simulink subsystem "BLDC_Motor_Sub2"  (R2020b)
settings: Solver=VariableStepAuto  StartTime=0.0  StopTime=10.0  RelTol=1e-3
libraries: fl_lib x29, nesl_utility x9, ee_lib x1
settings Model: Creator=Chrille Skog  LastModifiedBy=Chrille Skog

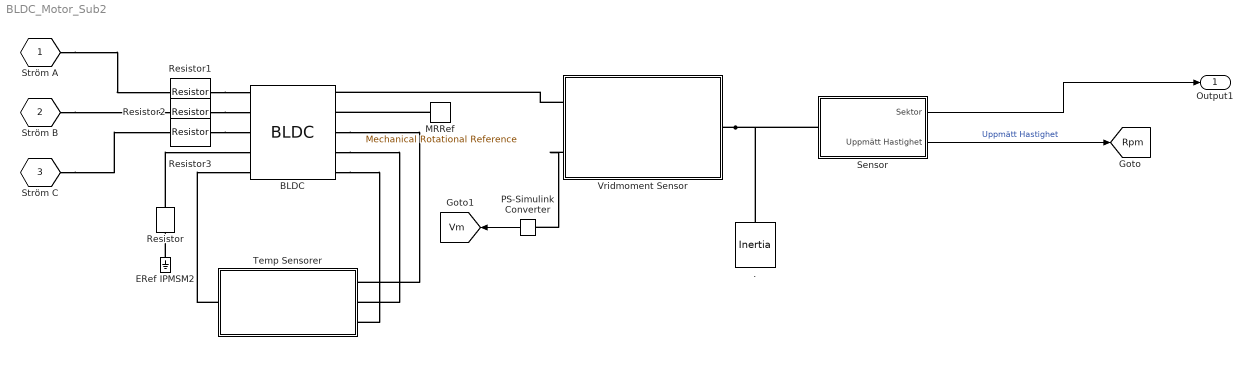
== system BLDC_Motor_Sub2 ==
  . : fl_lib/Mechanical/Rotational Elements/Inertia  inertia=2 kg*m^2  num_ports=foundation.enum.numPorts2.one  w_specify=off  w_priority=High  w=0 rpm  w_nominal_specify=off  w_nominal_unit=rad/s  w_nominal_value=1  t_specify=off  t_priority=High  t=0 N*m  t_nominal_specify=off  t_nominal_unit=N*m  t_nominal_value=1
      settings: SourceProductName=Foundation Library
  BLDC : ee_lib/Electromechanical/Permanent Magnet/BLDC  winding_type=ee.enum.statorconnection.wye  rotor_param=ee.enum.pmsm.backemf.trapezoidflux  pm_flux_linkage=0.05 Wb  theta_constant=120/3 deg  emf_max=9.6 V  DphiDtheta_tab=[0, -.1528, -.1528, .1528, .1528, 0] Wb/rad  back_emf_tab=[0, -9.6, -9.6, 9.6, 9.6, 0] V  rotor_angle_tab=[0, 7.5, 22.5, 37.5, 52.5, 60] deg  w_meas=600 rpm  nPolePairs=3  stator_param=ee.enum.statorparam.LdLqL0  machine_param=ee.enum.dqparameterization.constant  Ld=0.00022 H  Lq=0.00022 H  idVec=[-200, 0, 200] A  iqVec=[-200, 0, 200] A  LdMatrix=0.00022 * ones(3, 3) H  LqMatrix=0.00022 * ones(3, 3) H  L0=0.00016 H  Ls=0.0002 H  Lm=0 H  Ms=0.00002 H  Rs=0.0013 Ohm  zero_sequence=ee.enum.park.zerosequence.include  J=0 kg*m^2  lam=0.1 N*m/(rad/s)  axes_param=ee.enum.rotorangle.qaxis  i_d_specify=off  i_d_priority=None  i_d=0 A  i_d_nominal_specify=off  i_d_nominal_unit=A  i_d_nominal_value=1  i_q_specify=off  i_q_priority=None  i_q=0 A  i_q_nominal_specify=off  i_q_nominal_unit=A  i_q_nominal_value=1  torque_specify=off  torque_priority=None  torque=0 N*m  torque_nominal_specify=off  torque_nominal_unit=N*m  torque_nominal_value=1  angular_velocity_specify=off  angular_velocity_priority=High  angular_velocity=0 rpm  angular_velocity_nominal_specify=off  angular_velocity_nominal_unit=rpm  angular_velocity_nominal_value=1  angular_position_specify=off  angular_position_priority=High  angular_position=0 deg  angular_position_nominal_specify=off  angular_position_nominal_unit=deg  angular_position_nominal_value=1  loss_param=ee.enum.ironloss.none  losses_oc=[0, 0, 0] W  losses_sc=[0, 0, 0] W  f_losses=60 Hz  Isc_losses=95 A  Tmeas=298.15 K  alpha=3.93e-3 1/K  alpha_flux=-0.001 1/K  stator_thermal_mass=100 J/K  rotor_thermal_mass=200 J/K  Rm_percent_rotor=90  Rd_percent_rotor=30  temperatureA_specify=off  temperatureA_priority=High  temperatureA=25 degC  temperatureA_nominal_specify=off  temperatureA_nominal_unit=degC  temperatureA_nominal_value=1  temperatureB_specify=off  temperatureB_priority=High  temperatureB=25 degC  temperatureB_nominal_specify=off  temperatureB_nominal_unit=degC  temperatureB_nominal_value=1  temperatureC_specify=off  temperatureC_priority=High  temperatureC=25 degC  temperatureC_nominal_specify=off  temperatureC_nominal_unit=degC  temperatureC_nominal_value=1  temperatureR_specify=off  temperatureR_priority=High  temperatureR=25 degC  temperatureR_nominal_specify=off  temperatureR_nominal_unit=degC  temperatureR_nominal_value=1
      settings: SourceProductBaseCode=PS  InternalSimscapePortConfiguration="{\"Bottom\":[],\"Left\":[{\"id\":\"a\",\"label\":\"a\",\"type\":\"foundation.electrical.electrical\"},{\"id\":\"b\",\"label\":\"b\",\"type\":\"foundation.electrical.electrical\"},{\"id\":\"c\",\"label\":\"c\",\"type\":\"foundation.electrical.electrical\"},{\"id\":\"n\",\"label\":\"n\",\"type\":\"foundation.electrical.electrical\"},{\"id\":\"HR\",\"label\":\"HR\",\"type\":\"foundation.thermal.thermal\"}],\"Right\":[{\"id\":\"R\",\"label\":\"R\",\"type\":\"foundation.mechanical.rotational.rotational\"},{\"id\":\"C\",\"label\":\"C\",\"type\":\"foundation.mechanical.rotational.rotational\"},{\"id\":\"HA\",\"label\":\"HA\",\"type\":\"foundation.thermal.thermal\"},{\"id\":\"HB\",\"label\":\"HB\",\"type\":\"foundation.thermal.thermal\"},{\"id\":\"HC\",\"label\":\"HC\",\"type\":\"foundation.thermal.thermal\"}],\"Top\":[]}"
  ERef IPMSM2 : fl_lib/Electrical/Electrical Elements/Electrical Reference
  MRRef : fl_lib/Mechanical/Rotational Elements/Mechanical Rotational Reference
  PS-Simulink Converter : nesl_utility/PS-Simulink Converter  PhysicalDomain=network_engine_domain  SubClassName=ps_output  LeftPortType=input  RightPortType=output  PseudoPeriodic=off  Frequencies=[]  Unit=inherit  AffineConversion=off
  Resistor : fl_lib/Electrical/Electrical Elements/Resistor  R=1e9 Ohm  i_specify=off  i_priority=None  i=0 A  i_nominal_specify=off  i_nominal_unit=A  i_nominal_value=1  v_specify=off  v_priority=None  v=0 V  v_nominal_specify=off  v_nominal_unit=V  v_nominal_value=1
  Resistor1 : fl_lib/Electrical/Electrical Elements/Resistor  R=0 Ohm  i_specify=off  i_priority=None  i=0 A  i_nominal_specify=off  i_nominal_unit=A  i_nominal_value=1  v_specify=off  v_priority=None  v=0 V  v_nominal_specify=off  v_nominal_unit=V  v_nominal_value=1
  Resistor2 : fl_lib/Electrical/Electrical Elements/Resistor  R=0 Ohm  i_specify=off  i_priority=None  i=0 A  i_nominal_specify=off  i_nominal_unit=A  i_nominal_value=1  v_specify=off  v_priority=None  v=0 V  v_nominal_specify=off  v_nominal_unit=V  v_nominal_value=1
  Resistor3 : fl_lib/Electrical/Electrical Elements/Resistor  R=0 Ohm  i_specify=off  i_priority=None  i=0 A  i_nominal_specify=off  i_nominal_unit=A  i_nominal_value=1  v_specify=off  v_priority=None  v=0 V  v_nominal_specify=off  v_nominal_unit=V  v_nominal_value=1
  Sensor : Subsystem
  Temp Sensorer : Subsystem
  Vridmoment Sensor : Subsystem
  Ström A : PMIOPort  Tag=PMCPort  Side=Left
  Ström B : PMIOPort  Tag=PMCPort  Port=2  Side=Left
  Ström C : PMIOPort  Tag=PMCPort  Port=3  Side=Left
  Output1 : Outport
  tag scope: Rpm=global, Vm=global
  wires:
  Sensor/1(Sektor) -> Output1/1
  Sensor/2(Uppmätt Hastighet) -> [Rpm]  "Uppmätt Hastighet"
  PS-Simulink Converter/1 -> [Vm]
  connections:
  Vridmoment Sensor/RConn1 -- ./LConn1 -- Sensor/LConn1
  Ström B/RConn1 -- Resistor2/LConn1
  Resistor/LConn1 -- BLDC/LConn4
  Vridmoment Sensor/LConn1 -- BLDC/RConn1
  MRRef/LConn1 -- BLDC/RConn2
  BLDC/RConn4 -- Temp Sensorer/LConn2
  BLDC/RConn3 -- Temp Sensorer/LConn1
  Temp Sensorer/RConn1 -- BLDC/LConn5
  BLDC/RConn5 -- Temp Sensorer/LConn3
  ERef IPMSM2/LConn1 -- Resistor/RConn1
  Ström C/RConn1 -- Resistor3/LConn1
  Ström A/RConn1 -- Resistor1/LConn1
  Vridmoment Sensor/LConn2 -- PS-Simulink Converter/LConn1
  Resistor1/RConn1 -- BLDC/LConn1
  Resistor2/RConn1 -- BLDC/LConn2
  Resistor3/RConn1 -- BLDC/LConn3

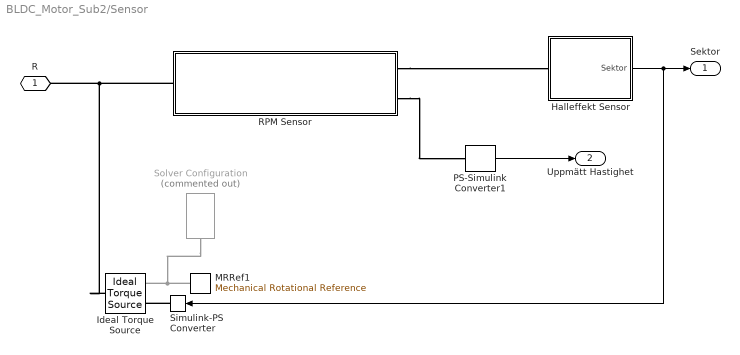
== system BLDC_Motor_Sub2/Sensor ==
  Halleffekt Sensor : Subsystem
  Ideal Torque Source : fl_lib/Mechanical/Mechanical Sources/Ideal Torque Source
  MRRef1 : fl_lib/Mechanical/Rotational Elements/Mechanical Rotational Reference
  PS-Simulink Converter1 : nesl_utility/PS-Simulink Converter  PhysicalDomain=network_engine_domain  SubClassName=ps_output  LeftPortType=input  RightPortType=output  PseudoPeriodic=off  Frequencies=[]  Unit=rpm  AffineConversion=off
  RPM Sensor : Subsystem
  Simulink-PS Converter : nesl_utility/Simulink-PS Converter  PhysicalDomain=network_engine_domain  SubClassName=ps_input  LeftPortType=input  RightPortType=output  PseudoPeriodic=off  Frequencies=[]  NoiseDistribution=none  NoiseParameters=[]  Unit=N*m  AffineConversion=off  FilteringAndDerivatives=provide  SimscapeFilterOrder=1  InputFilterTimeConstant=0.001  UdotUserProvided=0
  Solver Configuration : nesl_utility/Solver Configuration  Commented=on  PhysicalDomain=network_engine_domain  SubClassName=solver  LeftPortType=input  RightPortType=generic  Tones=[]  Harmonics=[]  SimulateNoise=off  Profile=off  UseLocalSampling=off  EnableSwitchedLinearOptims=on  FrequencyDomain=off  UseCCode=off  RelTol=0.001  AbsTol=1e-06  MinStep=1e-09  ToWorkspace=off  RevertToSquareIcSolve=off  NumHomotopyIterations=100  PhasorMode=off  PhasorModeNumHarmonics=1  DoDC=off  ResidualTolerance=1e-09  UseLocalSolver=on  LocalSolverChoice=NE_BACKWARD_EULER_ADVANCER  LocalSolverSampleTime=0.001  DoFixedCost=on  MaxNonlinIter=2  MaxModeIter=2  ComputeImpulses=off  ImpulseIterations=2  LinearAlgebra=auto  EquationFormulation=NE_TIME_EF  DelaysMemoryBudget=1024  AutomaticFiltering=on  FilteringTimeConstant=0.001  PartitionStorageMethod=AS_NEEDED  PartitionMemoryBudget=1024  PartitionMethod=FAST
  R : PMIOPort  Side=Left
  Sektor : Outport
  Uppmätt Hastighet : Outport  Port=2
  wires:
  PS-Simulink Converter1/1 -> Uppmätt Hastighet/1
  Halleffekt Sensor/1(Sektor) -> Simulink-PS Converter/1, Sektor/1
  connections:
  RPM Sensor/LConn1 -- R/RConn1 -- Ideal Torque Source/LConn1
  RPM Sensor/RConn2 -- PS-Simulink Converter1/LConn1
  RPM Sensor/RConn1 -- Halleffekt Sensor/LConn1
  Solver Configuration/RConn1 -- MRRef1/LConn1 -- Ideal Torque Source/RConn2
  Simulink-PS Converter/RConn1 -- Ideal Torque Source/RConn1

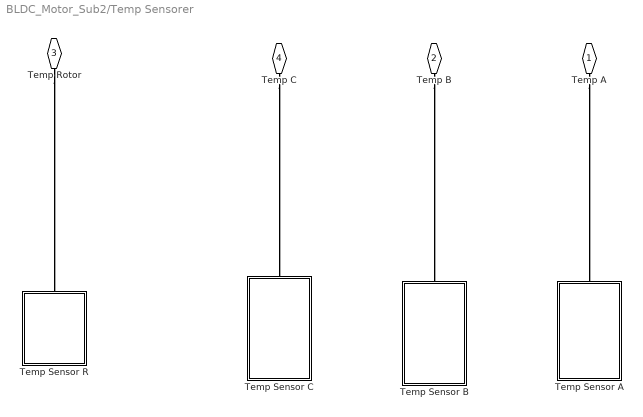
== system BLDC_Motor_Sub2/Temp Sensorer ==
  Temp Sensor A : Subsystem
  Temp Sensor B : Subsystem
  Temp Sensor C : Subsystem
  Temp Sensor R : Subsystem
  Temp A : PMIOPort  Side=Left
  Temp B : PMIOPort  Port=2  Side=Left
  "Temp Rotor " : PMIOPort  Port=3  Side=Right
  Temp C : PMIOPort  Port=4  Side=Left
  connections:
  Temp B/RConn1 -- Temp Sensor B/LConn1
  Temp A/RConn1 -- Temp Sensor A/LConn1
  Temp C/RConn1 -- Temp Sensor C/LConn1
  "Temp Rotor "/RConn1 -- Temp Sensor R/RConn1

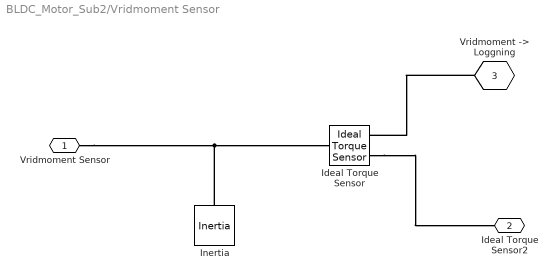
== system BLDC_Motor_Sub2/Vridmoment Sensor ==
  Ideal Torque Sensor : fl_lib/Mechanical/Mechanical Sensors/Ideal Torque Sensor
  Inertia : fl_lib/Mechanical/Rotational Elements/Inertia  inertia=0.01 kg*m^2  num_ports=foundation.enum.numPorts2.one  w_specify=off  w_priority=High  w=0 rad/s  w_nominal_specify=off  w_nominal_unit=rad/s  w_nominal_value=1  t_specify=off  t_priority=None  t=0 N*m  t_nominal_specify=off  t_nominal_unit=N*m  t_nominal_value=1
  Vridmoment Sensor : PMIOPort  Side=Left
  Ideal Torque Sensor2 : PMIOPort  Port=2  Side=Right
  "Vridmoment -> Loggning" : PMIOPort  Tag=PMCPort  Port=3  Side=Left
  connections:
  "Vridmoment -> Loggning"/RConn1 -- Ideal Torque Sensor/RConn2
  Ideal Torque Sensor/RConn1 -- Ideal Torque Sensor2/RConn1
  Vridmoment Sensor/RConn1 -- Ideal Torque Sensor/LConn1 -- Inertia/LConn1

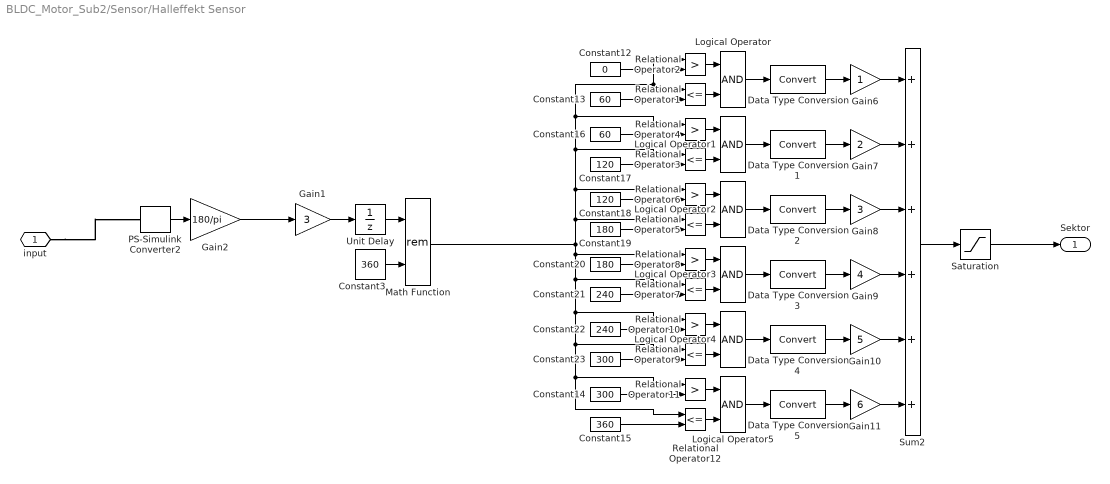
== system BLDC_Motor_Sub2/Sensor/Halleffekt Sensor ==
  Constant12 : Constant  Value=0
  Constant13 : Constant  Value=60
  Constant14 : Constant  Value=300
  Constant15 : Constant  Value=360
  Constant16 : Constant  Value=60
  Constant17 : Constant  Value=120
  Constant18 : Constant  Value=120
  Constant19 : Constant  Value=180
  Constant20 : Constant  Value=180
  Constant21 : Constant  Value=240
  Constant22 : Constant  Value=240
  Constant23 : Constant  Value=300
  Constant3 : Constant  Value=360
  Data Type Conversion{,1..5} (6 alike) : DataTypeConversion  SaturateOnIntegerOverflow=on  RndMeth=Zero
  Gain1 : Gain  Gain=3
  Gain10 : Gain  Gain=5  SaturateOnIntegerOverflow=on  OutDataTypeStr=Inherit: Same as input  ParamDataTypeStr=Inherit: Same as input
  Gain11 : Gain  Gain=6  SaturateOnIntegerOverflow=on  OutDataTypeStr=Inherit: Same as input  ParamDataTypeStr=Inherit: Same as input
  Gain2 : Gain  Gain=180/pi
  Gain6 : Gain  SaturateOnIntegerOverflow=on  OutDataTypeStr=Inherit: Same as input  ParamDataTypeStr=Inherit: Same as input
  Gain7 : Gain  Gain=2  SaturateOnIntegerOverflow=on  OutDataTypeStr=Inherit: Same as input  ParamDataTypeStr=Inherit: Same as input
  Gain8 : Gain  Gain=3  SaturateOnIntegerOverflow=on  OutDataTypeStr=Inherit: Same as input  ParamDataTypeStr=Inherit: Same as input
  Gain9 : Gain  Gain=4  SaturateOnIntegerOverflow=on  OutDataTypeStr=Inherit: Same as input  ParamDataTypeStr=Inherit: Same as input
  Logical Operator{,1..5} (6 alike) : Logic
  Math Function : Math  Operator=rem  SignedPower=on  SaturateOnIntegerOverflow=on
  PS-Simulink Converter2 : nesl_utility/PS-Simulink Converter  PhysicalDomain=network_engine_domain  SubClassName=ps_output  LeftPortType=input  RightPortType=output  PseudoPeriodic=off  Frequencies=[]  Unit=rad  AffineConversion=off
  Relational Operator{1,3,5,7,9,12} (6 alike) : RelationalOperator  Operator=<=  RndMeth=Nearest  InputSameDT=on
  Relational Operator{2,4,6,8,10..11} (6 alike) : RelationalOperator  Operator=>  RndMeth=Nearest  InputSameDT=on
  Saturation : Saturate  UpperLimit=6  LowerLimit=1
  Sum2 : Sum  Inputs=++++++  InputSameDT=on  SaturateOnIntegerOverflow=on  OutDataTypeStr=Inherit: Same as first input
  Unit Delay : UnitDelay  SampleTime=5.0e-5  HasFrameUpgradeWarning=on
  input : PMIOPort  Side=Left
  Sektor : Outport
  wires:
  Constant12/1 -> Relational Operator2/2
  Gain2/1 -> Gain1/1
  Math Function/1 -> Relational Operator2/1, Relational Operator1/1, Relational Operator4/1, Relational Operator3/1, Relational Operator6/1, Relational Operator5/1, Relational Operator12/1, Relational Operator11/1, Relational Operator9/1, Relational Operator10/1, Relational Operator7/1, Relational Operator8/1
  Relational Operator8/1 -> Logical Operator3/1
  Data Type Conversion5/1 -> Gain11/1
  Relational Operator7/1 -> Logical Operator3/2
  Logical Operator5/1 -> Data Type Conversion5/1
  Constant20/1 -> Relational Operator8/2
  Data Type Conversion1/1 -> Gain7/1
  Data Type Conversion2/1 -> Gain8/1
  Logical Operator2/1 -> Data Type Conversion2/1
  Constant18/1 -> Relational Operator6/2
  Relational Operator3/1 -> Logical Operator1/2
  Relational Operator4/1 -> Logical Operator1/1
  Logical Operator3/1 -> Data Type Conversion3/1
  Relational Operator9/1 -> Logical Operator4/2
  Data Type Conversion4/1 -> Gain10/1
  Relational Operator2/1 -> Logical Operator/1
  Relational Operator1/1 -> Logical Operator/2
  Sum2/1 -> Saturation/1
  Logical Operator/1 -> Data Type Conversion/1
  Constant19/1 -> Relational Operator5/2
  Constant16/1 -> Relational Operator4/2
  Constant17/1 -> Relational Operator3/2
  Relational Operator5/1 -> Logical Operator2/2
  Relational Operator6/1 -> Logical Operator2/1
  Gain10/1 -> Sum2/5
  Data Type Conversion3/1 -> Gain9/1
  Logical Operator1/1 -> Data Type Conversion1/1
  Relational Operator12/1 -> Logical Operator5/2
  Logical Operator4/1 -> Data Type Conversion4/1
  Constant21/1 -> Relational Operator7/2
  Constant22/1 -> Relational Operator10/2
  Gain8/1 -> Sum2/3
  Gain7/1 -> Sum2/2
  Data Type Conversion/1 -> Gain6/1
  Gain6/1 -> Sum2/1
  Relational Operator10/1 -> Logical Operator4/1
  PS-Simulink Converter2/1 -> Gain2/1
  Constant23/1 -> Relational Operator9/2
  Relational Operator11/1 -> Logical Operator5/1
  Constant13/1 -> Relational Operator1/2
  Constant3/1 -> Math Function/2
  Constant14/1 -> Relational Operator11/2
  Gain1/1 -> Unit Delay/1
  Gain9/1 -> Sum2/4
  Unit Delay/1 -> Math Function/1
  Gain11/1 -> Sum2/6
  Constant15/1 -> Relational Operator12/2
  Saturation/1 -> Sektor/1
  connections:
  input/RConn1 -- PS-Simulink Converter2/LConn1

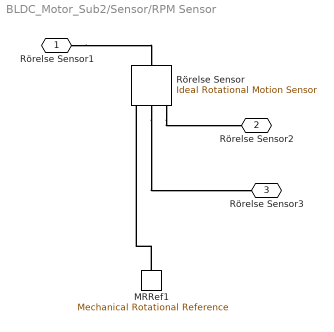
== system BLDC_Motor_Sub2/Sensor/RPM Sensor ==
  MRRef1 : fl_lib/Mechanical/Rotational Elements/Mechanical Rotational Reference
  Rörelse Sensor : fl_lib/Mechanical/Mechanical Sensors/Ideal Rotational Motion Sensor  wrap_angle=simscape.enum.onoff.off  offset=0 deg
      settings: SourceProductName=Foundation Library
  Rörelse Sensor1 : PMIOPort  Side=Left
  Rörelse Sensor2 : PMIOPort  Port=2  Side=Right
  Rörelse Sensor3 : PMIOPort  Port=3  Side=Right
  connections:
  Rörelse Sensor/RConn3 -- Rörelse Sensor2/RConn1
  MRRef1/LConn1 -- Rörelse Sensor/RConn1
  Rörelse Sensor1/RConn1 -- Rörelse Sensor/LConn1
  Rörelse Sensor/RConn2 -- Rörelse Sensor3/RConn1

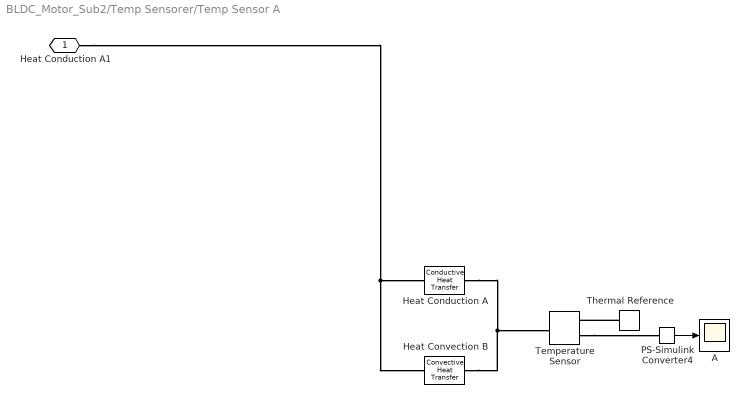
== system BLDC_Motor_Sub2/Temp Sensorer/Temp Sensor A ==
  A : Scope
  Heat Conduction A : fl_lib/Thermal/Thermal Elements/Conductive Heat Transfer  area=0.002 m^2  thickness=0.1 m  th_cond=80 W/(m*K)  T_specify=off  T_priority=None  T=0 K  T_nominal_specify=off  T_nominal_unit=K  T_nominal_value=1  Q_specify=off  Q_priority=None  Q=0 J/s  Q_nominal_specify=off  Q_nominal_unit=J/s  Q_nominal_value=1
      settings: SourceProductName=Foundation Library
  Heat Convection B : fl_lib/Thermal/Thermal Elements/Convective Heat Transfer  area=0.02 m^2  heat_tr_coeff=200 W/(m^2 * K)  T_specify=off  T_priority=None  T=0 K  T_nominal_specify=off  T_nominal_unit=K  T_nominal_value=1  Q_specify=off  Q_priority=None  Q=0 J/s  Q_nominal_specify=off  Q_nominal_unit=J/s  Q_nominal_value=1
      settings: SourceProductName=Foundation Library
  PS-Simulink Converter4 : nesl_utility/PS-Simulink Converter  PhysicalDomain=network_engine_domain  SubClassName=ps_output  LeftPortType=input  RightPortType=output  PseudoPeriodic=off  Frequencies=[]  Unit=K  AffineConversion=off
  Temperature Sensor : fl_lib/Thermal/Thermal Sensors/Temperature Sensor
      settings: SourceProductName=Foundation Library
  Thermal Reference : fl_lib/Thermal/Thermal Elements/Thermal Reference
  Heat Conduction A1 : PMIOPort  Side=Left
  wires:
  PS-Simulink Converter4/1 -> A/1
  connections:
  Thermal Reference/LConn1 -- Temperature Sensor/RConn1
  Temperature Sensor/RConn2 -- PS-Simulink Converter4/LConn1
  Heat Conduction A1/RConn1 -- Heat Conduction A/RConn1 -- Heat Convection B/RConn1
  Heat Convection B/LConn1 -- Temperature Sensor/LConn1 -- Heat Conduction A/LConn1

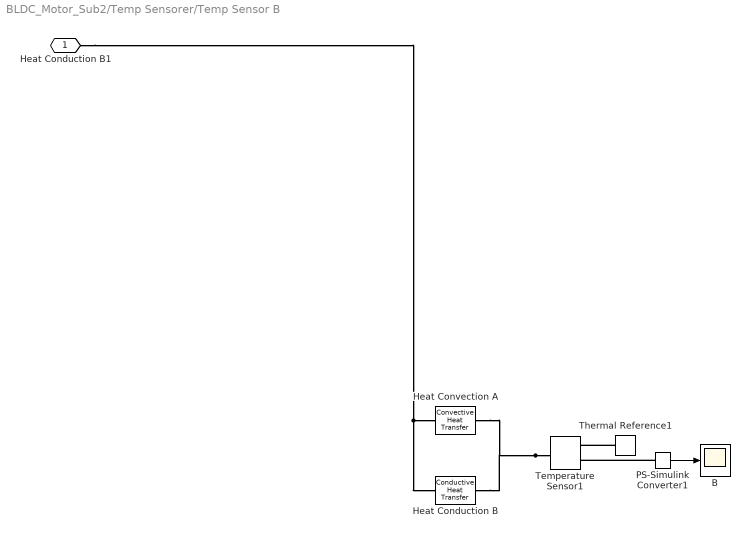
== system BLDC_Motor_Sub2/Temp Sensorer/Temp Sensor B ==
  B : Scope
  Heat Convection A : fl_lib/Thermal/Thermal Elements/Convective Heat Transfer  area=0.02 m^2  heat_tr_coeff=200 W/(m^2 * K)  T_specify=off  T_priority=None  T=0 K  T_nominal_specify=off  T_nominal_unit=K  T_nominal_value=1  Q_specify=off  Q_priority=None  Q=0 J/s  Q_nominal_specify=off  Q_nominal_unit=J/s  Q_nominal_value=1
      settings: SourceProductName=Foundation Library
  Heat Conduction B : fl_lib/Thermal/Thermal Elements/Conductive Heat Transfer  area=0.002 m^2  thickness=0.1 m  th_cond=80 W/(m*K)  T_specify=off  T_priority=None  T=0 K  T_nominal_specify=off  T_nominal_unit=K  T_nominal_value=1  Q_specify=off  Q_priority=None  Q=0 J/s  Q_nominal_specify=off  Q_nominal_unit=J/s  Q_nominal_value=1
      settings: SourceProductName=Foundation Library
  PS-Simulink Converter1 : nesl_utility/PS-Simulink Converter  PhysicalDomain=network_engine_domain  SubClassName=ps_output  LeftPortType=input  RightPortType=output  PseudoPeriodic=off  Frequencies=[]  Unit=K  AffineConversion=off
  Temperature Sensor1 : fl_lib/Thermal/Thermal Sensors/Temperature Sensor
      settings: SourceProductName=Foundation Library
  Thermal Reference1 : fl_lib/Thermal/Thermal Elements/Thermal Reference
  Heat Conduction B1 : PMIOPort  Side=Left
  wires:
  PS-Simulink Converter1/1 -> B/1
  connections:
  Heat Conduction B1/RConn1 -- Heat Convection A/RConn1 -- Heat Conduction B/RConn1
  Temperature Sensor1/LConn1 -- Heat Convection A/LConn1 -- Heat Conduction B/LConn1
  Thermal Reference1/LConn1 -- Temperature Sensor1/RConn1
  PS-Simulink Converter1/LConn1 -- Temperature Sensor1/RConn2

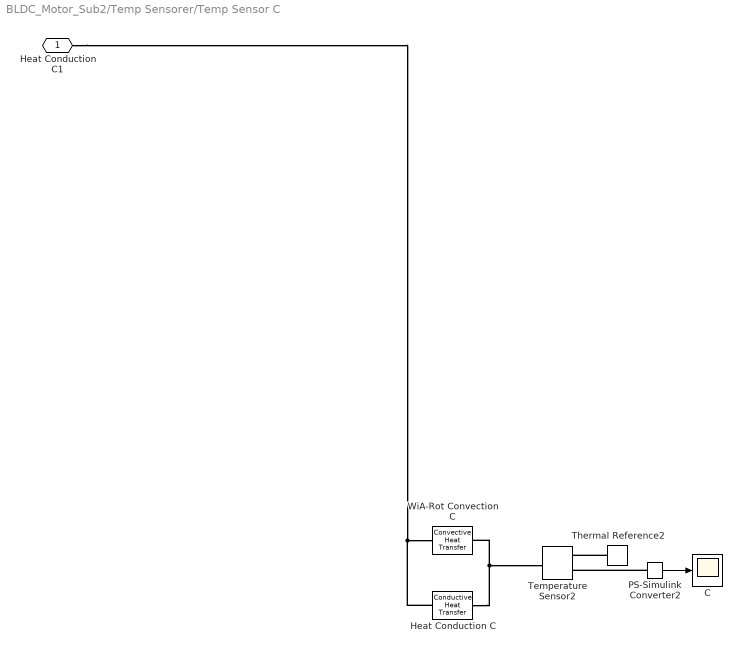
== system BLDC_Motor_Sub2/Temp Sensorer/Temp Sensor C ==
  C : Scope
  Heat Conduction C : fl_lib/Thermal/Thermal Elements/Conductive Heat Transfer  area=0.002 m^2  thickness=0.1 m  th_cond=80 W/(m*K)  T_specify=off  T_priority=None  T=0 K  T_nominal_specify=off  T_nominal_unit=K  T_nominal_value=1  Q_specify=off  Q_priority=None  Q=0 J/s  Q_nominal_specify=off  Q_nominal_unit=J/s  Q_nominal_value=1
      settings: SourceProductName=Foundation Library
  PS-Simulink Converter2 : nesl_utility/PS-Simulink Converter  PhysicalDomain=network_engine_domain  SubClassName=ps_output  LeftPortType=input  RightPortType=output  PseudoPeriodic=off  Frequencies=[]  Unit=K  AffineConversion=off
  Temperature Sensor2 : fl_lib/Thermal/Thermal Sensors/Temperature Sensor
      settings: SourceProductName=Foundation Library
  Thermal Reference2 : fl_lib/Thermal/Thermal Elements/Thermal Reference
  WiA-Rot Convection C : fl_lib/Thermal/Thermal Elements/Convective Heat Transfer  area=0.02 m^2  heat_tr_coeff=200 W/(m^2 * K)  T_specify=off  T_priority=None  T=0 K  T_nominal_specify=off  T_nominal_unit=K  T_nominal_value=1  Q_specify=off  Q_priority=None  Q=0 J/s  Q_nominal_specify=off  Q_nominal_unit=J/s  Q_nominal_value=1
      settings: SourceProductName=Foundation Library
  Heat Conduction C1 : PMIOPort  Side=Left
  wires:
  PS-Simulink Converter2/1 -> C/1
  connections:
  Heat Conduction C/RConn1 -- WiA-Rot Convection C/RConn1 -- Heat Conduction C1/RConn1
  Thermal Reference2/LConn1 -- Temperature Sensor2/RConn1
  Heat Conduction C/LConn1 -- WiA-Rot Convection C/LConn1 -- Temperature Sensor2/LConn1
  PS-Simulink Converter2/LConn1 -- Temperature Sensor2/RConn2

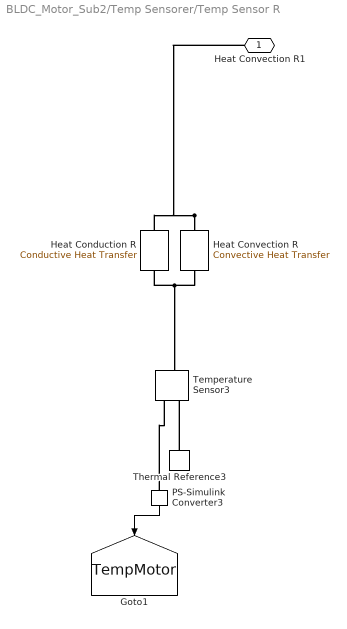
== system BLDC_Motor_Sub2/Temp Sensorer/Temp Sensor R ==
  Heat Conduction R : fl_lib/Thermal/Thermal Elements/Conductive Heat Transfer  area=0.002 m^2  thickness=0.1 m  th_cond=80 W/(m*K)  T_specify=off  T_priority=None  T=0 K  T_nominal_specify=off  T_nominal_unit=K  T_nominal_value=1  Q_specify=off  Q_priority=None  Q=0 J/s  Q_nominal_specify=off  Q_nominal_unit=J/s  Q_nominal_value=1
      settings: SourceProductName=Foundation Library
  Heat Convection R : fl_lib/Thermal/Thermal Elements/Convective Heat Transfer  area=0.02 m^2  heat_tr_coeff=200 W/(m^2 * K)  T_specify=off  T_priority=None  T=0 K  T_nominal_specify=off  T_nominal_unit=K  T_nominal_value=1  Q_specify=off  Q_priority=None  Q=0 J/s  Q_nominal_specify=off  Q_nominal_unit=J/s  Q_nominal_value=1
      settings: SourceProductName=Foundation Library
  PS-Simulink Converter3 : nesl_utility/PS-Simulink Converter  PhysicalDomain=network_engine_domain  SubClassName=ps_output  LeftPortType=input  RightPortType=output  PseudoPeriodic=off  Frequencies=[]  Unit=K  AffineConversion=off
  Temperature Sensor3 : fl_lib/Thermal/Thermal Sensors/Temperature Sensor
      settings: SourceProductName=Foundation Library
  Thermal Reference3 : fl_lib/Thermal/Thermal Elements/Thermal Reference
  Heat Convection R1 : PMIOPort  Side=Right
  tag scope: TempMotor=global
  wires:
  PS-Simulink Converter3/1 -> [TempMotor]
  connections:
  Heat Convection R/RConn1 -- Heat Conduction R/RConn1 -- Heat Convection R1/RConn1
  PS-Simulink Converter3/LConn1 -- Temperature Sensor3/RConn2
  Heat Convection R/LConn1 -- Heat Conduction R/LConn1 -- Temperature Sensor3/LConn1
  Thermal Reference3/LConn1 -- Temperature Sensor3/RConn1
